simulink model "Valve_PHY_TestBed"  (R2012b)
settings: Solver=FixedStepDiscrete  StartTime=0.0  StopTime=1  FixedStep=1  RelTol=1e-3
undefined symbols (not defined in the file): MWS
libraries: Lib_Turbo_ValvePHY_TMATS x1
settings Model: Creator=jwchapm2  LastModifiedBy=jwchapm2

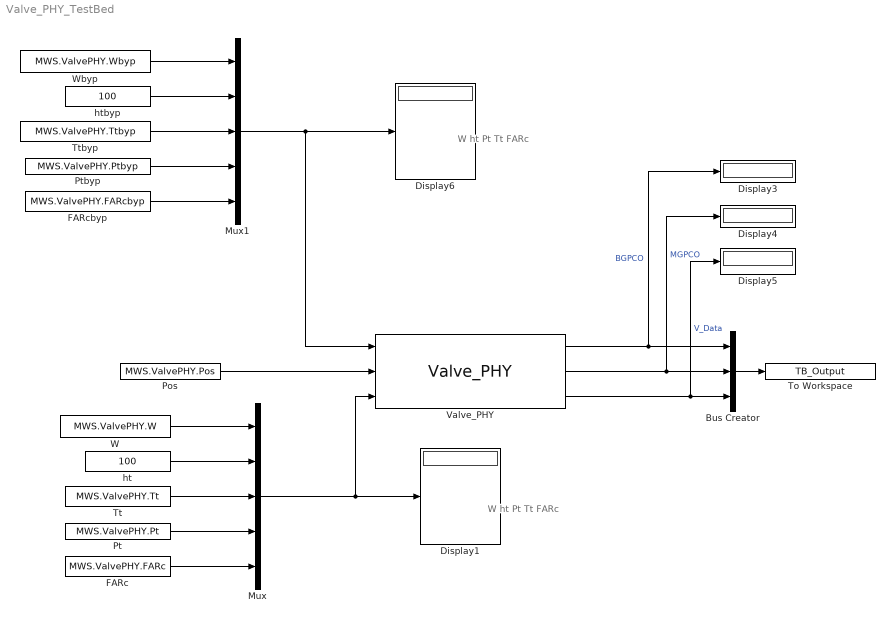
== system Valve_PHY_TestBed ==
  note: W
      | ht
      | Pt
      | Tt
      | FARc
  note: W
      | ht
      | Pt
      | Tt
      | FARc
  Bus Creator : BusCreator  Inputs=3
  Display{1,3..6} (5 alike) : Display
  FARc : Constant  Value=MWS.ValvePHY.FARc
  FARcbyp : Constant  Value=MWS.ValvePHY.FARcbyp
  Mux : Mux  Inputs=5
  Mux1 : Mux  Inputs=5
  Pos : Constant  Value=MWS.ValvePHY.Pos
  Pt : Constant  Value=MWS.ValvePHY.Pt
  Ptbyp : Constant  Value=MWS.ValvePHY.Ptbyp
  To Workspace : ToWorkspace  VariableName=TB_Output  SampleTime=-1
  Tt : Constant  Value=MWS.ValvePHY.Tt
  Ttbyp : Constant  Value=MWS.ValvePHY.Ttbyp
  Valve_PHY : Lib_Turbo_ValvePHY_TMATS/Valve_PHY  s_V_AeVLV_M=200  s_V_AeBYP_M=200  s_V_AeTH_M=167  X_V_FARVec_M=[1 10]  T_V_RtVec_M=[0 .99]  Y_V_TtVec_M=[1 10]  T_V_gammaArray_M=[1.4 1.4; 1.4 1.4]
  W : Constant  Value=MWS.ValvePHY.W
  Wbyp : Constant  Value=MWS.ValvePHY.Wbyp
  ht : Constant  Value=100
  htbyp : Constant  Value=100
  wires:
  Pos/1 -> Valve_PHY/2
  W/1 -> Mux/1
  FARc/1 -> Mux/5
  Tt/1 -> Mux/3
  Pt/1 -> Mux/4
  Mux/1 -> Valve_PHY/3, Display1/1
  Valve_PHY/1 -> Display3/1, Bus Creator/1  "BGPCO"
  Valve_PHY/2 -> Display4/1, Bus Creator/2  "MGPCO"
  Valve_PHY/3 -> Display5/1, Bus Creator/3  "V_Data"
  Bus Creator/1 -> To Workspace/1
  ht/1 -> Mux/2
  Wbyp/1 -> Mux1/1
  FARcbyp/1 -> Mux1/5
  Ttbyp/1 -> Mux1/3
  Ptbyp/1 -> Mux1/4
  Mux1/1 -> Valve_PHY/1, Display6/1
  htbyp/1 -> Mux1/2
